simulink model "TimeDelayed_KF"  (Simulink 7.0)
settings: Solver=ode5  StartTime=0.0  StopTime=10.0  FixedStep=0.1  RelTol=1e-3
undefined symbols (not defined in the file or in its folder): DiscIntNeverNeededParam
libraries: simulink x1
settings Model: Creator=mish_hr  LastModifiedBy=mish_hr  ExtModeAutoUpdateStatusClock=off

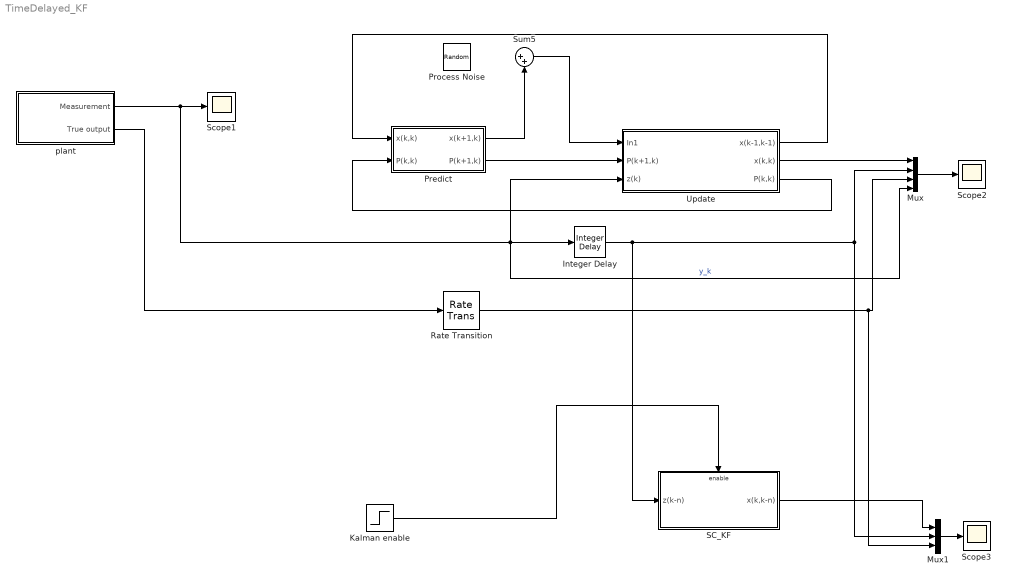
== system TimeDelayed_KF ==
  Integer Delay : simulink/Discrete/Integer Delay  vinit=0.0  samptime=0.1  NumDelays=5
  Kalman enable : Step  Time=0.5  SampleTime=0
  Mux : Mux
  Mux1 : Mux  Inputs=3
  Predict : Subsystem
  Process Noise : RandomNumber  Variance=0.0001
  Rate Transition : RateTransition  OutPortSampleTime=0.1
  SC_KF : Subsystem
  Scope1 : Scope
      settings: TimeRange=10
  Scope2 : Scope
      settings: TimeRange=10
  Scope3 : Scope
      settings: TimeRange=10  SaveName=ScopeData3
  Sum5 : Sum  Inputs=|++  OutDataType=sfix(16)  OutScaling=2^0  SampleTime=0.1
  Update : Subsystem
  plant : Subsystem
  wires:
  plant/1(Measurement) -> Scope1/1, Integer Delay/1, Update/3(z(k)), Mux/4  "y_k"
  Update/1(x(k-1,k-1)) -> Predict/1(x(k,k))
  Mux/1 -> Scope2/1
  Update/3(P(k,k)) -> Predict/2(P(k,k))
  Predict/1(x(k+1,k)) -> Sum5/2
  Update/2(x(k,k)) -> Mux/1
  Sum5/1 -> Update/1(In1)
  Predict/2(P(k+1,k)) -> Update/2(P(k+1,k))
  plant/2(True output) -> Rate Transition/1
  Rate Transition/1 -> Mux/3, Mux1/3
  Integer Delay/1 -> Mux/2, Mux1/2, SC_KF/1(z(k-n))
  SC_KF/1(x(k,k-n)) -> Mux1/1
  Mux1/1 -> Scope3/1
  Kalman enable/1 -> SC_KF/Enable

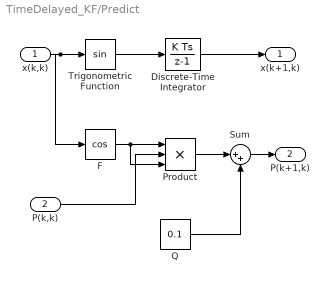
== system TimeDelayed_KF/Predict ==
  x(k,k) : Inport
  P(k,k) : Inport  Port=2
  Discrete-Time Integrator : DiscreteIntegrator  InitialCondition=2  SampleTime=0.1  OutDataType=sfix(16)  OutScaling=2^0  ICPrevOutput=DiscIntNeverNeededParam  ICPrevScaledInput=DiscIntNeverNeededParam
  F : Trigonometry  Operator=cos  SampleTime=0.1
  Product : Product  Inputs=3  OutDataType=sfix(16)  OutScaling=2^0  SampleTime=0.1  RndMeth=Zero
  Q : Constant  Value=0.1  OutDataType=sfix(16)  OutScaling=2^0
  Sum : Sum  Inputs=|++  OutDataType=sfix(16)  OutScaling=2^0  SampleTime=0.1
  Trigonometric Function : Trigonometry  SampleTime=0.1
  x(k+1,k) : Outport
  P(k+1,k) : Outport  Port=2
  wires:
  Trigonometric Function/1 -> Discrete-Time Integrator/1
  F/1 -> Product/1, Product/3
  P(k,k)/1 -> Product/2
  Product/1 -> Sum/1
  Q/1 -> Sum/2
  Discrete-Time Integrator/1 -> x(k+1,k)/1
  x(k,k)/1 -> Trigonometric Function/1, F/1
  Sum/1 -> P(k+1,k)/1

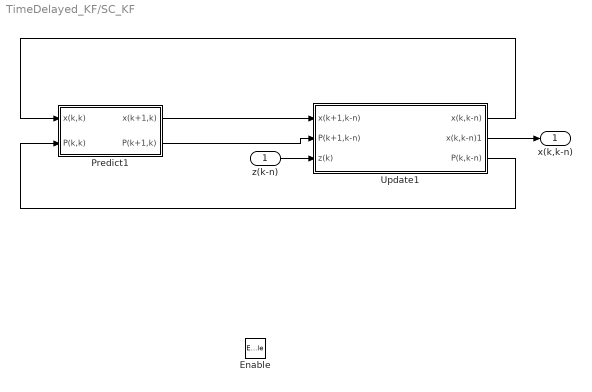
== system TimeDelayed_KF/SC_KF ==
  z(k-n) : Inport
  Enable : EnablePort
  Predict1 : Subsystem
  Update1 : Subsystem
  x(k,k-n) : Outport
  wires:
  Update1/1(x(k,k-n)) -> Predict1/1(x(k,k))
  Update1/3(P(k,k-n)) -> Predict1/2(P(k,k))
  Predict1/1(x(k+1,k)) -> Update1/1(x(k+1,k-n))
  Predict1/2(P(k+1,k)) -> Update1/2(P(k+1,k-n))
  z(k-n)/1 -> Update1/3(z(k))
  Update1/2(x(k,k-n)1) -> x(k,k-n)/1

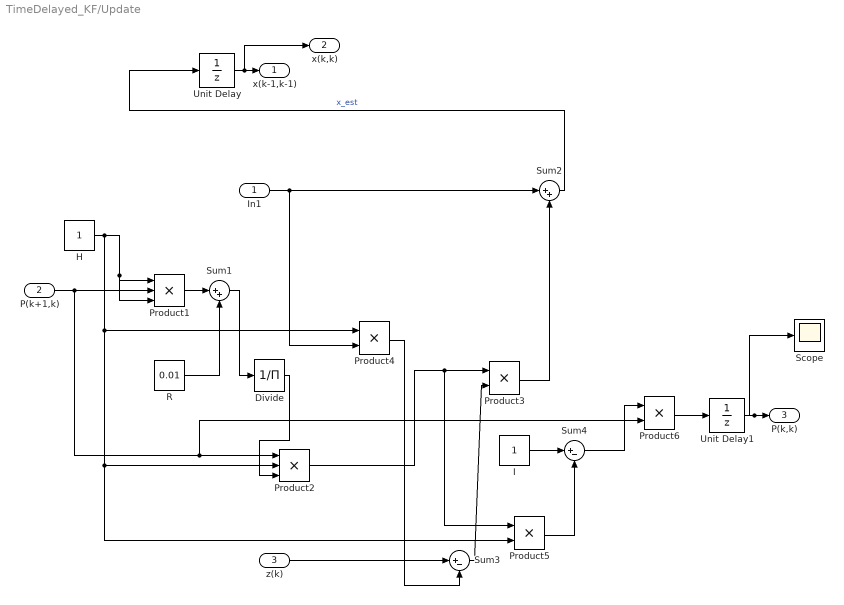
== system TimeDelayed_KF/Update ==
  In1 : Inport
  P(k+1,k) : Inport  Port=2
  z(k) : Inport  Port=3
  Divide : Product  Inputs=/  OutDataType=sfix(16)  OutScaling=2^-10
  H : Constant  OutDataType=sfix(16)  OutScaling=2^0
  I : Constant  OutDataType=sfix(16)  OutScaling=2^0
  Product1 : Product  Inputs=3  OutDataType=sfix(16)  OutScaling=2^0  SampleTime=0.1  RndMeth=Zero
  Product2 : Product  Inputs=3  OutDataType=sfix(16)  OutScaling=2^0  SampleTime=0.1  RndMeth=Zero
  Product3 : Product  OutDataType=sfix(16)  OutScaling=2^0  SampleTime=0.1  RndMeth=Zero
  Product4 : Product  OutDataType=sfix(16)  OutScaling=2^0  RndMeth=Zero
  Product5 : Product  OutDataType=sfix(16)  OutScaling=2^0  RndMeth=Zero
  Product6 : Product  OutDataType=sfix(16)  OutScaling=2^0  SampleTime=0.1  RndMeth=Zero
  R : Constant  Value=0.01  OutDataType=sfix(16)  OutScaling=2^0
  Scope : Scope
      settings: SaveName=ScopeData2
  Sum1 : Sum  Inputs=|++  OutDataType=sfix(16)  OutScaling=2^0
  Sum2 : Sum  Inputs=|++  OutDataType=sfix(16)  OutScaling=2^0  SampleTime=0.1
  Sum3 : Sum  Inputs=|+-  OutDataType=sfix(16)  OutScaling=2^0
  Sum4 : Sum  Inputs=|+-  OutDataType=sfix(16)  OutScaling=2^0
  Unit Delay : UnitDelay  X0=3  SampleTime=0.1
  Unit Delay1 : UnitDelay  X0=2  SampleTime=0.1
  x(k-1,k-1) : Outport
  x(k,k) : Outport  Port=2
  P(k,k) : Outport  Port=3
  wires:
  P(k+1,k)/1 -> Product1/2, Product2/1, Product6/2
  Sum4/1 -> Product6/1
  In1/1 -> Product4/2, Sum2/1
  Product5/1 -> Sum4/2
  I/1 -> Sum4/1
  Sum2/1 -> Unit Delay/1  "x_est"
  Product3/1 -> Sum2/2
  Sum3/1 -> Product3/2
  Product4/1 -> Sum3/2
  Product2/1 -> Product3/1, Product5/1
  R/1 -> Sum1/2
  Product1/1 -> Sum1/1
  H/1 -> Product1/1, Product1/3, Product4/1, Product2/2, Product5/2
  z(k)/1 -> Sum3/1
  Unit Delay/1 -> x(k-1,k-1)/1, x(k,k)/1
  Product6/1 -> Unit Delay1/1
  Unit Delay1/1 -> P(k,k)/1, Scope/1
  Sum1/1 -> Divide/1
  Divide/1 -> Product2/3

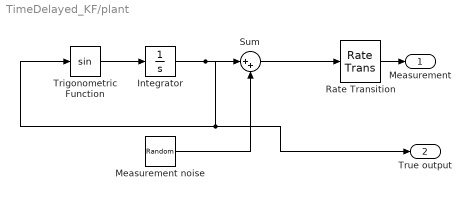
== system TimeDelayed_KF/plant ==
  Integrator : Integrator  InitialCondition=0.1
  Measurement noise : RandomNumber  Variance=0.05
  Rate Transition : RateTransition  OutPortSampleTime=0.1
  Sum : Sum  Inputs=|++  OutDataType=sfix(16)  OutScaling=2^0
  Trigonometric Function : Trigonometry
  Measurement : Outport
  True output : Outport  Port=2
  wires:
  Integrator/1 -> Sum/1, Trigonometric Function/1, True output/1
  Sum/1 -> Rate Transition/1
  Rate Transition/1 -> Measurement/1
  Trigonometric Function/1 -> Integrator/1
  Measurement noise/1 -> Sum/2

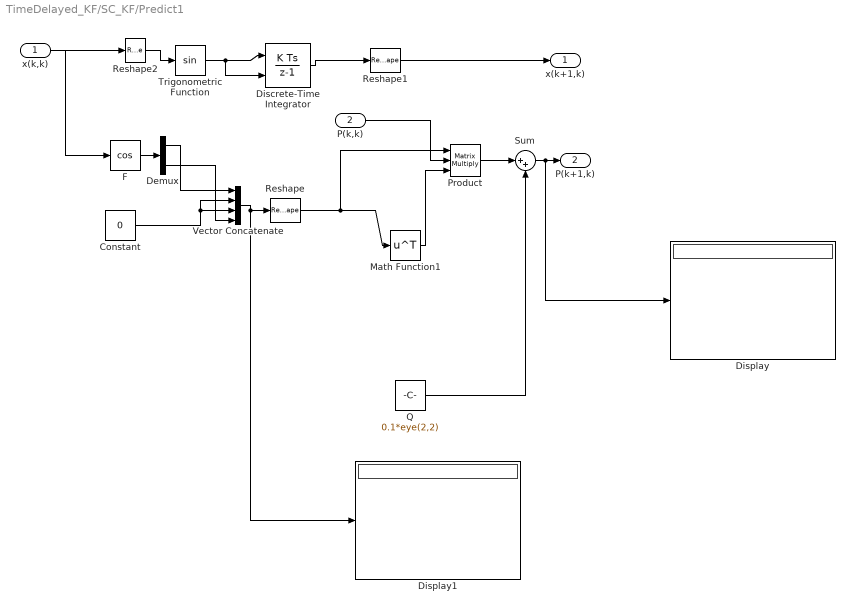
== system TimeDelayed_KF/SC_KF/Predict1 ==
  x(k,k) : Inport
  P(k,k) : Inport  Port=2
  Constant : Constant  Value=0  OutDataType=sfix(16)  OutScaling=2^0
  Demux : Demux  Outputs=2
  Discrete-Time Integrator : DiscreteIntegrator  InitialConditionSource=external  InitialCondition=[1; 1]  SampleTime=0.1  OutDataType=sfix(16)  OutScaling=2^0  ICPrevOutput=DiscIntNeverNeededParam  ICPrevScaledInput=DiscIntNeverNeededParam
  Display : Display
  Display1 : Display
  F : Trigonometry  Operator=cos  SampleTime=0.1
  Math Function1 : Math  Operator=transpose  OutDataType=sfix(16)  OutScaling=2^0  SaturateOnIntegerOverflow=on
  Product : Product  Inputs=3  Multiplication=Matrix(*)  OutDataType=sfix(16)  OutScaling=2^0  SampleTime=0.1  RndMeth=Zero
  Q : Constant  Value=0.1*eye(2,2)  OutDataType=sfix(16)  OutScaling=2^0
  Reshape : Reshape  OutputDimensionality=Customize  OutputDimensions=[2,2]
  Reshape1 : Reshape  OutputDimensionality=Customize  OutputDimensions=[2,1]
  Reshape2 : Reshape  OutputDimensionality=Customize  OutputDimensions=[2,1]
  Sum : Sum  Inputs=|++  OutDataType=sfix(16)  OutScaling=2^0  SampleTime=0.1
  Trigonometric Function : Trigonometry  SampleTime=0.1
  Vector Concatenate : Concatenate  NumInputs=4  Mode=Vector
  x(k+1,k) : Outport
  P(k+1,k) : Outport  Port=2
  wires:
  Sum/1 -> P(k+1,k)/1, Display/1
  Discrete-Time Integrator/1 -> Reshape1/1
  Q/1 -> Sum/2
  Product/1 -> Sum/1
  F/1 -> Demux/1
  Trigonometric Function/1 -> Discrete-Time Integrator/1, Discrete-Time Integrator/2
  Demux/1 -> Vector Concatenate/1
  Constant/1 -> Vector Concatenate/2, Vector Concatenate/3
  P(k,k)/1 -> Product/2
  Vector Concatenate/1 -> Display1/1, Reshape/1
  Reshape1/1 -> x(k+1,k)/1
  x(k,k)/1 -> F/1, Reshape2/1
  Reshape2/1 -> Trigonometric Function/1
  Math Function1/1 -> Product/3
  Demux/2 -> Vector Concatenate/4
  Reshape/1 -> Product/1, Math Function1/1

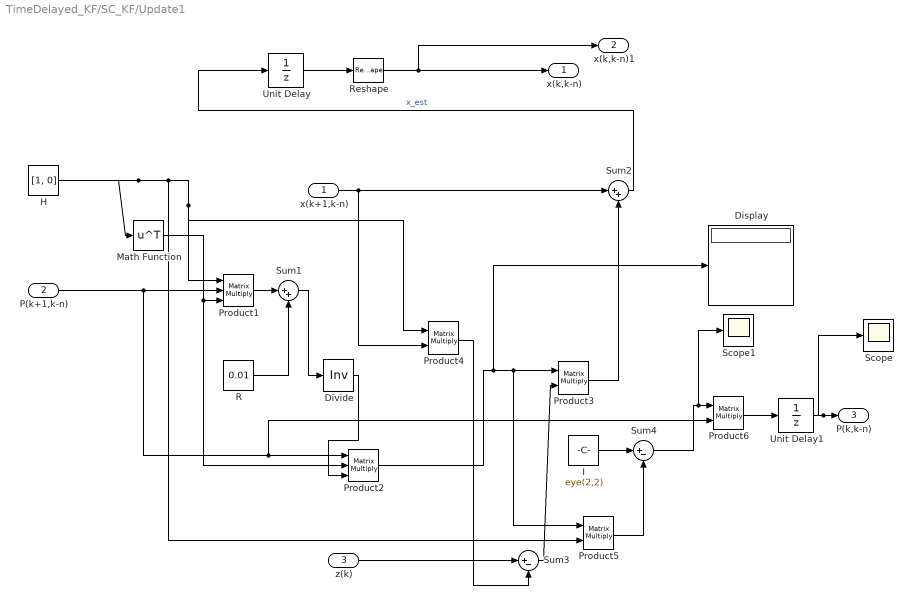
== system TimeDelayed_KF/SC_KF/Update1 ==
  x(k+1,k-n) : Inport
  P(k+1,k-n) : Inport  Port=2
  z(k) : Inport  Port=3
  Display : Display
  Divide : Product  Inputs=/  Multiplication=Matrix(*)  OutDataType=sfix(16)  OutScaling=2^-10
  H : Constant  Value=[1, 0]  VectorParams1D=off  OutDataType=sfix(16)  OutScaling=2^0
  I : Constant  Value=eye(2,2)  OutDataType=sfix(16)  OutScaling=2^0
  Math Function : Math  Operator=transpose  OutDataType=sfix(16)  OutScaling=2^0  SaturateOnIntegerOverflow=on
  Product1 : Product  Inputs=3  Multiplication=Matrix(*)  OutDataType=sfix(16)  OutScaling=2^0  SampleTime=0.1  RndMeth=Zero
  Product2 : Product  Inputs=3  Multiplication=Matrix(*)  OutDataType=sfix(16)  OutScaling=2^0  SampleTime=0.1  RndMeth=Zero
  Product3 : Product  Multiplication=Matrix(*)  OutDataType=sfix(16)  OutScaling=2^0  SampleTime=0.1  RndMeth=Zero
  Product4 : Product  Multiplication=Matrix(*)  OutDataType=sfix(16)  OutScaling=2^0  RndMeth=Zero
  Product5 : Product  Multiplication=Matrix(*)  OutDataType=sfix(16)  OutScaling=2^0  RndMeth=Zero
  Product6 : Product  Multiplication=Matrix(*)  OutDataType=sfix(16)  OutScaling=2^0  SampleTime=0.1  RndMeth=Zero
  R : Constant  Value=0.01  OutDataType=sfix(16)  OutScaling=2^0
  Reshape : Reshape  OutputDimensionality=Customize  OutputDimensions=[2,1]
  Scope : Scope
      settings: SaveName=ScopeData2
  Scope1 : Scope
      settings: SaveName=ScopeData4
  Sum1 : Sum  Inputs=|++  OutDataType=sfix(16)  OutScaling=2^0
  Sum2 : Sum  Inputs=|++  OutDataType=sfix(16)  OutScaling=2^0  SampleTime=0.1
  Sum3 : Sum  Inputs=|+-  OutDataType=sfix(16)  OutScaling=2^0
  Sum4 : Sum  Inputs=|+-  OutDataType=sfix(16)  OutScaling=2^0
  Unit Delay : UnitDelay  X0=[1;1]  SampleTime=0.1
  Unit Delay1 : UnitDelay  X0=2*ones(2,2)  SampleTime=0.1
  x(k,k-n) : Outport
  x(k,k-n)1 : Outport  Port=2
  P(k,k-n) : Outport  Port=3
  wires:
  Divide/1 -> Product2/3
  Sum1/1 -> Divide/1
  Unit Delay1/1 -> Scope/1, P(k,k-n)/1
  Product6/1 -> Unit Delay1/1
  Unit Delay/1 -> Reshape/1
  z(k)/1 -> Sum3/1
  H/1 -> Math Function/1, Product1/1, Product4/1, Product5/2
  Product1/1 -> Sum1/1
  R/1 -> Sum1/2
  Product2/1 -> Product5/1, Product3/1, Display/1
  Product4/1 -> Sum3/2
  Sum3/1 -> Product3/2
  Product3/1 -> Sum2/2
  Sum2/1 -> Unit Delay/1  "x_est"
  I/1 -> Sum4/1
  Product5/1 -> Sum4/2
  x(k+1,k-n)/1 -> Sum2/1, Product4/2
  Sum4/1 -> Product6/1, Scope1/1
  P(k+1,k-n)/1 -> Product6/2, Product2/1, Product1/2
  Math Function/1 -> Product1/3, Product2/2
  Reshape/1 -> x(k,k-n)1/1, x(k,k-n)/1
